simulink model "power_machines_Hatch"  (R2014a)
settings: Solver=ode23tb  SolverMode=SingleTasking  StartTime=0.0  StopTime=60  RelTol=1e-4
undefined symbols (not defined in the file or in its folder): A, B, C, Continuous, Dd, Ka, Ke, Kf, SeVe1, SeVe2, spsAC1AModel, Ta, Te, Tf, VAmax, VAmin, Ve0, Ve1, Ve2, Vfe0, VRmax, VRmin
undefined symbols (not defined in the file): Tb, Tc
libraries: sps_avr x19, powerlib x16, simulink_extras x4
(part 2 of 2)

== system power_machines_Hatch/EXCITATION1/AC1A/AC1A/Model/Continuous/Vaminmax ==
  note: Vfe0/Ka
  note: Vfe0
  note: Vfe0
  note: 0
  note: Vfe0
  u : Inport
  Gain1 : Gain  Gain=1/Ta  SaturateOnIntegerOverflow=on  OutDataTypeStr=Inherit: Same as input  ParamDataTypeStr=Inherit: Same as input
  Gain2 : Gain  Gain=Ka  SaturateOnIntegerOverflow=on  OutDataTypeStr=Inherit: Same as input  ParamDataTypeStr=Inherit: Same as input
  Integrator : Integrator  InitialCondition=Vfe0  LimitOutput=on  UpperSaturationLimit=VAmax  LowerSaturationLimit=VAmin
  Sum : Sum  Inputs=|+-  SaturateOnIntegerOverflow=on  InputSameDT=on  OutDataTypeStr=Inherit: Same as first input
  y : Outport
  wires:
  u/1 -> Gain2/1
  Sum/1 -> Gain1/1
  Integrator/1 -> y/1, Sum/2
  Gain2/1 -> Sum/1
  Gain1/1 -> Integrator/1

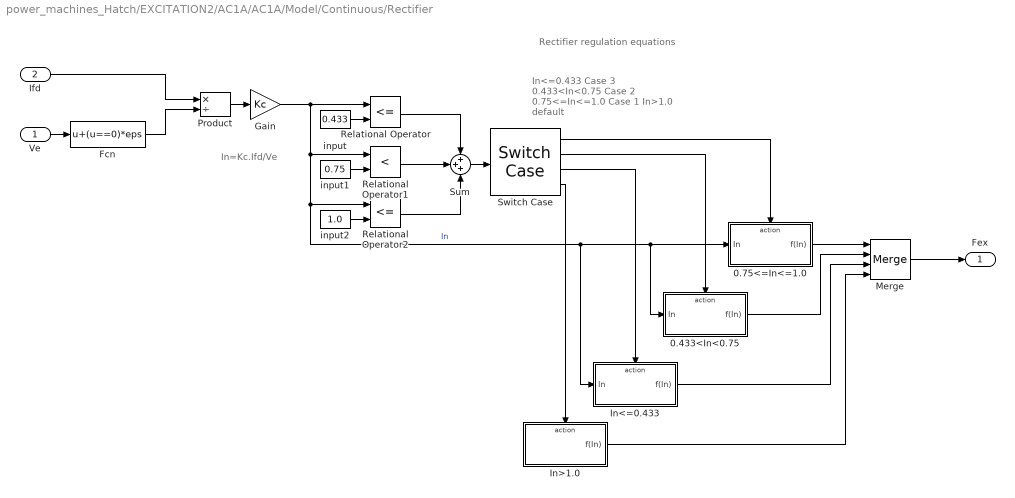
== system power_machines_Hatch/EXCITATION2/AC1A/AC1A/Model/Continuous/Rectifier ==
  note: In<=0.433        Case 3
      | 0.433<In<0.75 Case 2
      | 0.75<=In<=1.0 Case 1
      | In>1.0               default
  note: Rectifier regulation equations
  note: In=Kc.Ifd/Ve
  Ve : Inport
  Ifd : Inport  Port=2
  0.433<In<0.75 : Subsystem  TreatAsAtomicUnit=on
  0.75<=In<=1.0 : Subsystem  TreatAsAtomicUnit=on
  Fcn : Fcn  Expr=u+(u==0)*eps
  Gain : Gain  Gain=Kc  SaturateOnIntegerOverflow=on  OutDataTypeStr=Inherit: Same as input  ParamDataTypeStr=Inherit: Same as input
  In<=0.433 : Subsystem  TreatAsAtomicUnit=on
  In>1.0 : Subsystem  TreatAsAtomicUnit=on
  Merge : Merge  Inputs=4
  Product : Product  Inputs=*/  SaturateOnIntegerOverflow=on  RndMeth=Zero  InputSameDT=on  OutDataTypeStr=Inherit: Same as first input
  Relational Operator : RelationalOperator  Operator=<=  InputSameDT=on
  Relational Operator1 : RelationalOperator  Operator=<  InputSameDT=on
  Relational Operator2 : RelationalOperator  Operator=<=  InputSameDT=on
  Sum : Sum  Inputs=+++  AccumDataTypeStr=double  OutDataTypeStr=double  SaturateOnIntegerOverflow=on  InputSameDT=on
  Switch Case : SwitchCase  CaseConditions={1 2 3}
  input : Constant  Value=0.433
  input1 : Constant  Value=0.75
  input2 : Constant  Value=1.0
  Fex : Outport
  wires:
  Ve/1 -> Fcn/1
  Fcn/1 -> Product/2
  Ifd/1 -> Product/1
  Product/1 -> Gain/1
  Gain/1 -> Relational Operator2/1, 0.433<In<0.75/1(In), 0.75<=In<=1.0/1(In), In<=0.433/1(In), Relational Operator1/1, Relational Operator/1  "In"
  Merge/1 -> Fex/1
  0.75<=In<=1.0/1(f(In)) -> Merge/1
  0.433<In<0.75/1(f(In)) -> Merge/2
  In>1.0/1(f(In)) -> Merge/4
  In<=0.433/1(f(In)) -> Merge/3
  input1/1 -> Relational Operator1/2
  input2/1 -> Relational Operator2/2
  Relational Operator1/1 -> Sum/2
  Relational Operator/1 -> Sum/1
  Relational Operator2/1 -> Sum/3
  Sum/1 -> Switch Case/1
  Switch Case/1 -> 0.75<=In<=1.0/Action
  Switch Case/2 -> 0.433<In<0.75/Action
  Switch Case/3 -> In<=0.433/Action
  Switch Case/4 -> In>1.0/Action
  input/1 -> Relational Operator/2

== system power_machines_Hatch/EXCITATION2/AC1A/AC1A/Model/Continuous/Saturation Vx=Ve*Se[Ve] ==
  Ve : Inport
  Product : Product  SaturateOnIntegerOverflow=on  RndMeth=Zero  InputSameDT=on  OutDataTypeStr=Inherit: Same as first input
  Saturation : Lookup  InputValues=[0 Ve2 Ve1]  Table=[0 SeVe2 SeVe1]  SaturateOnIntegerOverflow=on
  Vx : Outport
  wires:
  Ve/1 -> Product/1, Saturation/1
  Saturation/1 -> Product/2
  Product/1 -> Vx/1

== system power_machines_Hatch/EXCITATION2/AC1A/AC1A/Model/Continuous/Transient Gain Reduction (Tc.s+1)//(Tb.s+1) ==
  In1 : Inport
  State Space : StateSpace  A=A  B=B  C=C  D=Dd  X0=X0
  Out1 : Outport  InitialOutput=0
  wires:
  State Space/1 -> Out1/1
  In1/1 -> State Space/1

== system power_machines_Hatch/EXCITATION2/AC1A/AC1A/Model/Continuous/Vaminmax ==
  note: Vfe0/Ka
  note: Vfe0
  note: Vfe0
  note: 0
  note: Vfe0
  u : Inport
  Gain1 : Gain  Gain=1/Ta  SaturateOnIntegerOverflow=on  OutDataTypeStr=Inherit: Same as input  ParamDataTypeStr=Inherit: Same as input
  Gain2 : Gain  Gain=Ka  SaturateOnIntegerOverflow=on  OutDataTypeStr=Inherit: Same as input  ParamDataTypeStr=Inherit: Same as input
  Integrator : Integrator  InitialCondition=Vfe0  LimitOutput=on  UpperSaturationLimit=VAmax  LowerSaturationLimit=VAmin
  Sum : Sum  Inputs=|+-  SaturateOnIntegerOverflow=on  InputSameDT=on  OutDataTypeStr=Inherit: Same as first input
  y : Outport
  wires:
  u/1 -> Gain2/1
  Sum/1 -> Gain1/1
  Integrator/1 -> y/1, Sum/2
  Gain2/1 -> Sum/1
  Gain1/1 -> Integrator/1

== system power_machines_Hatch/EXCITATION1/AC1A/AC1A/Model/Continuous/Rectifier/0.433<In<0.75 ==
  In : Inport
  Action Port : ActionPort  InitializeStates=reset  ActionType=case
  Math Function : Math  Operator=square  SaturateOnIntegerOverflow=on
  Math Function1 : Math  Operator=sqrt  SaturateOnIntegerOverflow=on
  Sum : Sum  Inputs=+-|  SaturateOnIntegerOverflow=on  InputSameDT=on  OutDataTypeStr=Inherit: Same as first input
  input2 : Constant  Value=0.75
  f(In) : Outport
  wires:
  Math Function1/1 -> f(In)/1
  In/1 -> Math Function/1
  Math Function/1 -> Sum/2
  input2/1 -> Sum/1
  Sum/1 -> Math Function1/1

== system power_machines_Hatch/EXCITATION1/AC1A/AC1A/Model/Continuous/Rectifier/0.75<=In<=1.0 ==
  In : Inport
  Action Port : ActionPort  InitializeStates=reset  ActionType=case
  Gain : Gain  Gain=1.732  SaturateOnIntegerOverflow=on  OutDataTypeStr=Inherit: Same as input  ParamDataTypeStr=Inherit: Same as input
  Sum : Sum  Inputs=+-|  SaturateOnIntegerOverflow=on  InputSameDT=on  OutDataTypeStr=Inherit: Same as first input
  input2 : Constant  Value=1.0
  f(In) : Outport
  wires:
  Gain/1 -> f(In)/1
  Sum/1 -> Gain/1
  input2/1 -> Sum/1
  In/1 -> Sum/2

== system power_machines_Hatch/EXCITATION1/AC1A/AC1A/Model/Continuous/Rectifier/In<=0.433 ==
  In : Inport
  Action Port : ActionPort  InitializeStates=reset  ActionType=case
  Gain : Gain  Gain=0.577  SaturateOnIntegerOverflow=on  OutDataTypeStr=Inherit: Same as input  ParamDataTypeStr=Inherit: Same as input
  Sum : Sum  Inputs=+-|  SaturateOnIntegerOverflow=on  InputSameDT=on  OutDataTypeStr=Inherit: Same as first input
  input2 : Constant  Value=1.0
  f(In) : Outport
  wires:
  Sum/1 -> f(In)/1
  input2/1 -> Sum/1
  Gain/1 -> Sum/2
  In/1 -> Gain/1

== system power_machines_Hatch/EXCITATION1/AC1A/AC1A/Model/Continuous/Rectifier/In>1.0 ==
  Action Port : ActionPort  InitializeStates=reset  ActionType=default
  input2 : Constant  Value=0
  f(In) : Outport  InitialOutput=0
  wires:
  input2/1 -> f(In)/1

== system power_machines_Hatch/EXCITATION2/AC1A/AC1A/Model/Continuous/Rectifier/0.433<In<0.75 ==
  In : Inport
  Action Port : ActionPort  InitializeStates=reset  ActionType=case
  Math Function : Math  Operator=square  SaturateOnIntegerOverflow=on
  Math Function1 : Math  Operator=sqrt  SaturateOnIntegerOverflow=on
  Sum : Sum  Inputs=+-|  SaturateOnIntegerOverflow=on  InputSameDT=on  OutDataTypeStr=Inherit: Same as first input
  input2 : Constant  Value=0.75
  f(In) : Outport
  wires:
  Math Function1/1 -> f(In)/1
  In/1 -> Math Function/1
  Math Function/1 -> Sum/2
  input2/1 -> Sum/1
  Sum/1 -> Math Function1/1

== system power_machines_Hatch/EXCITATION2/AC1A/AC1A/Model/Continuous/Rectifier/0.75<=In<=1.0 ==
  In : Inport
  Action Port : ActionPort  InitializeStates=reset  ActionType=case
  Gain : Gain  Gain=1.732  SaturateOnIntegerOverflow=on  OutDataTypeStr=Inherit: Same as input  ParamDataTypeStr=Inherit: Same as input
  Sum : Sum  Inputs=+-|  SaturateOnIntegerOverflow=on  InputSameDT=on  OutDataTypeStr=Inherit: Same as first input
  input2 : Constant  Value=1.0
  f(In) : Outport
  wires:
  Gain/1 -> f(In)/1
  Sum/1 -> Gain/1
  input2/1 -> Sum/1
  In/1 -> Sum/2

== system power_machines_Hatch/EXCITATION2/AC1A/AC1A/Model/Continuous/Rectifier/In<=0.433 ==
  In : Inport
  Action Port : ActionPort  InitializeStates=reset  ActionType=case
  Gain : Gain  Gain=0.577  SaturateOnIntegerOverflow=on  OutDataTypeStr=Inherit: Same as input  ParamDataTypeStr=Inherit: Same as input
  Sum : Sum  Inputs=+-|  SaturateOnIntegerOverflow=on  InputSameDT=on  OutDataTypeStr=Inherit: Same as first input
  input2 : Constant  Value=1.0
  f(In) : Outport
  wires:
  Sum/1 -> f(In)/1
  input2/1 -> Sum/1
  Gain/1 -> Sum/2
  In/1 -> Gain/1

== system power_machines_Hatch/EXCITATION2/AC1A/AC1A/Model/Continuous/Rectifier/In>1.0 ==
  Action Port : ActionPort  InitializeStates=reset  ActionType=default
  input2 : Constant  Value=0
  f(In) : Outport  InitialOutput=0
  wires:
  input2/1 -> f(In)/1
